simulink model "planof"  (R2014a)
settings: Solver=ode3  StartTime=0.0  StopTime=ts  FixedStep=tm  RelTol=1e-3
values from neighbouring files (symbols this model uses):
  AA = [0 1;-wn^2 -2*wn*xi]    [plfase.m]
  BB = [0;1]    [plfase.m]
  CC = eye(2)    [plfase.m]
  DD = [0;0]    [plfase.m]
  Q = 2    [plfase.m]
  X0 = [x10;x20]    [plfase.m]
settings Model: Creator=mau  LastModifiedBy=mau

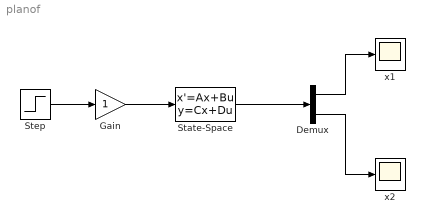
== system planof ==
  Demux : Demux  Outputs=2
  Gain : Gain
  State-Space : StateSpace  A=AA  B=BB  C=CC  D=DD  X0=X0
  Step : Step  Time=0  After=Q  SampleTime=0
  x1 : Scope
      settings: YMin=1  YMax=1.22
  x2 : Scope
      settings: YMin=-2  YMax=2.25
  wires:
  Step/1 -> Gain/1
  State-Space/1 -> Demux/1
  Demux/1 -> x1/1
  Demux/2 -> x2/1
  Gain/1 -> State-Space/1
